simulink model "asynchronous_motor_3phase_squirell_cage"  (R2017b)
settings: Solver=VariableStepAuto  StartTime=0.0  StopTime=100  RelTol=1e-3
values from neighbouring files (symbols this model uses):
  J = 1    [asynchronous_3phase_squirell_cage_parameters.m]
  Kr = Lm/Lr    (= 0.5)    [asynchronous_3phase_squirell_cage_parameters.m]
  Lm = 0.05    [asynchronous_3phase_squirell_cage_parameters.m]
  Lr = 0.1    [asynchronous_3phase_squirell_cage_parameters.m]
  Ls = 0.1    [asynchronous_3phase_squirell_cage_parameters.m]
  M = 0    [asynchronous_3phase_squirell_cage_parameters.m]
  Rs = 10    [asynchronous_3phase_squirell_cage_parameters.m]
  Tr = Lr/Rr    (= 0.01)    [asynchronous_3phase_squirell_cage_parameters.m]
  Z = 1    [asynchronous_3phase_squirell_cage_parameters.m]
settings Model: Creator=Алексей  LastModifiedBy=Алексей

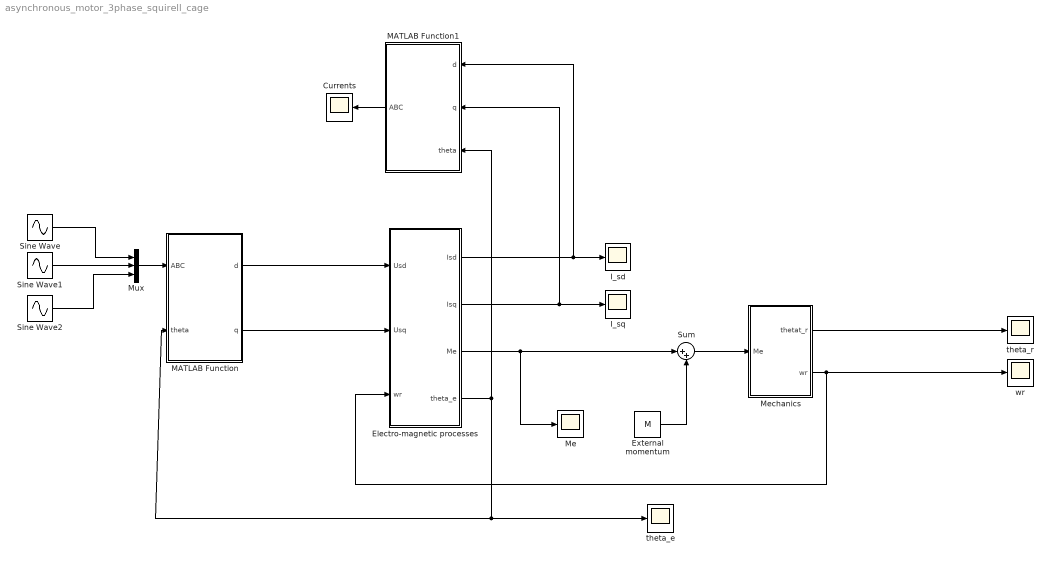
== system asynchronous_motor_3phase_squirell_cage ==
  Currents : Scope
  Electro-magnetic processes : Subsystem
  External momentum : Constant  Value=M
  I_sd : Scope
  I_sq : Scope
  MATLAB Function : MATLAB Function  TreatAsAtomicUnit=on
  MATLAB Function1 : MATLAB Function  TreatAsAtomicUnit=on
  Me : Scope
  Mechanics : Subsystem
  Mux : Mux  Inputs=3
  Sine Wave : Sin  Amplitude=220  Frequency=50  SampleTime=0
  Sine Wave1 : Sin  Amplitude=220  Frequency=50  Phase=-2*pi/3  SampleTime=0
  Sine Wave2 : Sin  Amplitude=220  Frequency=50  Phase=2*pi/3  SampleTime=0
  Sum : Sum  Inputs=|++
  theta_e : Scope
  theta_r : Scope
  wr : Scope
  wires:
  Mechanics/2(wr) -> wr/1, Electro-magnetic processes/3("wr ")
  Mechanics/1(thetat_r) -> theta_r/1
  MATLAB Function/1(d) -> Electro-magnetic processes/1(Usd)
  MATLAB Function/2(q) -> Electro-magnetic processes/2(Usq)
  Electro-magnetic processes/1(Isd) -> MATLAB Function1/1(d), I_sd/1
  Electro-magnetic processes/2(Isq) -> MATLAB Function1/2(q), I_sq/1
  Electro-magnetic processes/4(theta_e) -> MATLAB Function1/3(theta), MATLAB Function/2(theta), theta_e/1
  Electro-magnetic processes/3(Me) -> Sum/1, Me/1
  Mux/1 -> MATLAB Function/1(ABC)
  Sine Wave/1 -> Mux/1
  Sine Wave1/1 -> Mux/2
  Sine Wave2/1 -> Mux/3
  MATLAB Function1/1(ABC) -> Currents/1
  Sum/1 -> Mechanics/1(Me)
  External momentum/1 -> Sum/2

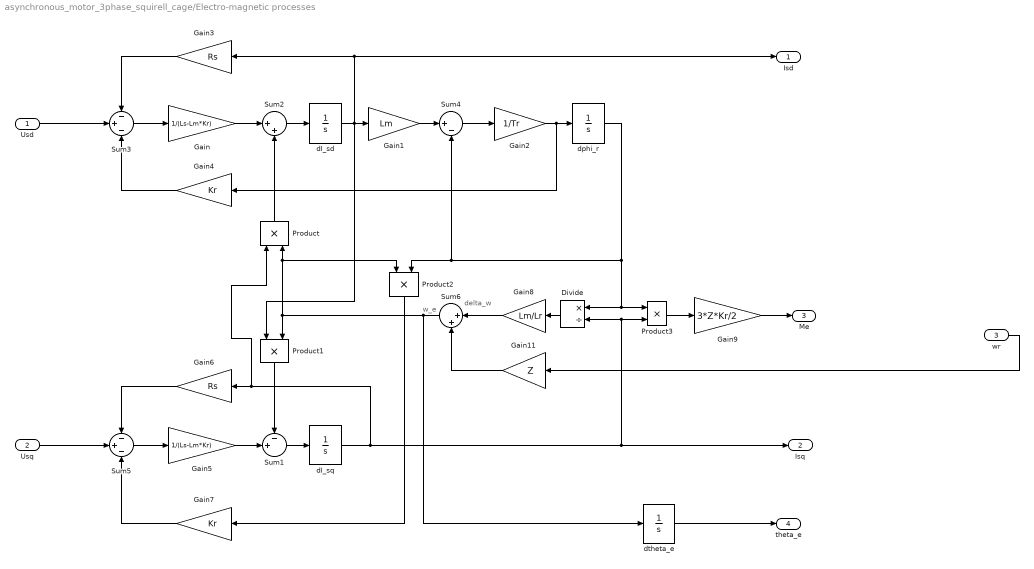
== system asynchronous_motor_3phase_squirell_cage/Electro-magnetic processes ==
  note: delta_w
  note: w_e
  Usd : Inport
  Usq : Inport  Port=2
  "wr " : Inport  Port=3
  Divide : Product  Inputs=*/
  Gain : Gain  Gain=1/(Ls-Lm*Kr)
  Gain1 : Gain  Gain=Lm
  Gain11 : Gain  Gain=Z
  Gain2 : Gain  Gain=1/Tr
  Gain3 : Gain  Gain=Rs
  Gain4 : Gain  Gain=Kr
  Gain5 : Gain  Gain=1/(Ls-Lm*Kr)
  Gain6 : Gain  Gain=Rs
  Gain7 : Gain  Gain=Kr
  Gain8 : Gain  Gain=Lm/Lr
  Gain9 : Gain  Gain=3*Z*Kr/2
  Product{,1..3} (4 alike) : Product
  Sum1 : Sum  Inputs=-+|
  Sum2 : Sum  Inputs=|++
  Sum3 : Sum  Inputs=-+-
  Sum4 : Sum  Inputs=|+-
  Sum5 : Sum  Inputs=-+-
  Sum6 : Sum  Inputs=|++
  dI_sd : Integrator  InitialCondition=0.01
  dI_sq : Integrator  InitialCondition=0.01
  dphi_r : Integrator  InitialCondition=0.01
  dtheta_e : Integrator  InitialCondition=0.01
  Isd : Outport
  Isq : Outport  Port=2
  Me : Outport  Port=3
  theta_e : Outport  Port=4
  wires:
  Usd/1 -> Sum3/2
  Gain1/1 -> Sum4/1
  Product3/1 -> Gain9/1
  Gain3/1 -> Sum3/1
  Sum3/1 -> Gain/1
  Gain8/1 -> Sum6/1
  Gain/1 -> Sum2/1
  Sum2/1 -> dI_sd/1
  Gain4/1 -> Sum3/3
  Sum4/1 -> Gain2/1
  Sum5/1 -> Gain5/1
  Product/1 -> Sum2/2
  "wr "/1 -> Gain11/1
  Gain9/1 -> Me/1
  Sum6/1 -> dtheta_e/1, Product2/1, Product/2, Product1/2
  Divide/1 -> Gain8/1
  dtheta_e/1 -> theta_e/1
  Gain7/1 -> Sum5/3
  Gain5/1 -> Sum1/2
  Gain11/1 -> Sum6/2
  Gain2/1 -> Gain4/1, dphi_r/1
  Sum1/1 -> dI_sq/1
  dI_sd/1 -> Product1/1, Isd/1, Gain3/1, Gain1/1
  dphi_r/1 -> Sum4/2, Product2/2, Divide/1, Product3/1
  Product1/1 -> Sum1/1
  Usq/1 -> Sum5/2
  dI_sq/1 -> Product/1, Gain6/1, Isq/1, Divide/2, Product3/2
  Gain6/1 -> Sum5/1
  Product2/1 -> Gain7/1

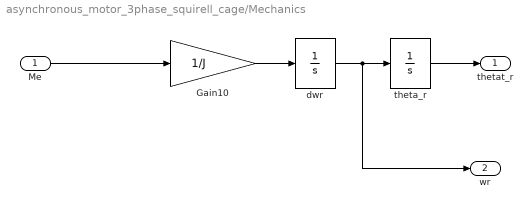
== system asynchronous_motor_3phase_squirell_cage/Mechanics ==
  Me : Inport
  Gain10 : Gain  Gain=1/J
  dwr : Integrator  InitialCondition=0.01
  theta_r : Integrator  InitialCondition=0.01
  thetat_r : Outport
  wr : Outport  Port=2
  wires:
  Gain10/1 -> dwr/1
  theta_r/1 -> thetat_r/1
  dwr/1 -> theta_r/1, wr/1
  Me/1 -> Gain10/1

== matlab function asynchronous_motor_3phase_squirell_cage/MATLAB Function1 ==
  data: d input; q input; ABC output; theta input
function ABC  = dq_ABC(d, q, theta)
A = d*cos(theta)-q*sin(theta);
B = sqrt(3)/2*(q*cos(theta)+d*sin(theta))-0.5*A;
C = -sqrt(3)/2*(q*cos(theta)+d*sin(theta))-0.5*A;

ABC=[A; B; C];

== matlab function asynchronous_motor_3phase_squirell_cage/MATLAB Function ==
  data: ABC input; d output; theta input; q output
function [d, q] = ABC_dq(ABC, theta)
A = ABC(1);
B = ABC(2);
C = ABC(3);

d = (B-C)/sqrt(3)*sin(theta)+A*cos(theta);
q = (B-C)/sqrt(3)*cos(theta)-A*sin(theta);
